simulink model "biomasaCambioEntrada"  (R2018a)
settings: Solver=VariableStepAuto  StartTime=0.0  StopTime=200  RelTol=1e-3
libraries: simulink x3
settings Model: Creator=Asus  LastModifiedBy=Asus
settings CodeAppCC: StateflowObjectComments=on

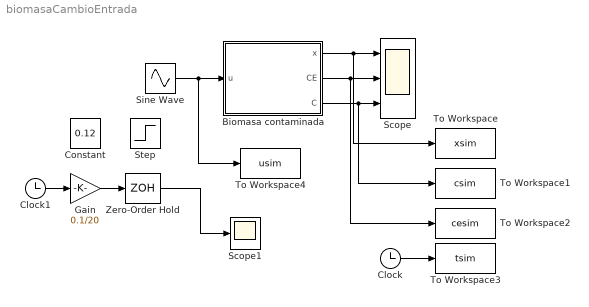
== system biomasaCambioEntrada ==
  Biomasa contaminada : Subsystem  mask(Modelo){par=[0.01,0.01,0.2,0.2,0.1,0.1,5,0.01,2], ci=[2,0,2]}
      mask prompts: par "[n, a, b, h, mu, r0, k0, r1, p]"; ci "[x0, c0, ce0]"
      mask help:
      | Modelo de concentración de contaminación en un ambiente
      | Entrada: contaminación
      | Salidas: biomasa de la población (x), concentración de toxina en el ambiente (Ce), cantidad de toxina en la biomasa de la población (C)
      mask init:
      | n  = par(1);
      | a  = par(2); 
      | b  = par(3);
      | h  = par(4);
      | mu = par(5); 
      | r0 = par(6); 
      | k0 = par(7); 
      | r1 = par(8); 
      | p  = par(9); 
      | x0 = ci(1);
      | c0 = ci(2);
      | ce0 = ci(3);
  Clock : Clock
  Clock1 : Clock
  Constant : Constant  Value=0.12
  Gain : Gain  Gain=0.1/20
  Scope : Scope  NumInputPorts=3
  Scope1 : Scope
  Sine Wave : Sin  Amplitude=0.5  Frequency=0.2  SampleTime=0
  Step : Step  Time=50  After=0.5  SampleTime=0
  To Workspace : ToWorkspace  VariableName=xsim  SampleTime=-1
      settings: Save2DSignal=2-D array (concatenate along first dimension)
  To Workspace1 : ToWorkspace  VariableName=csim  SampleTime=-1
      settings: Save2DSignal=2-D array (concatenate along first dimension)
  To Workspace2 : ToWorkspace  VariableName=cesim  SampleTime=-1
      settings: Save2DSignal=2-D array (concatenate along first dimension)
  To Workspace3 : ToWorkspace  VariableName=tsim  SampleTime=-1
  To Workspace4 : ToWorkspace  VariableName=usim  SampleTime=-1
  Zero-Order Hold : ZeroOrderHold  SampleTime=20
  wires:
  Biomasa contaminada/1(x) -> To Workspace/1, Scope/1
  Clock/1 -> To Workspace3/1
  Biomasa contaminada/2(CE) -> To Workspace2/1, Scope/2
  Biomasa contaminada/3(C) -> To Workspace1/1, Scope/3
  Gain/1 -> Zero-Order Hold/1
  Zero-Order Hold/1 -> Scope1/1
  Clock1/1 -> Gain/1
  Sine Wave/1 -> To Workspace4/1, Biomasa contaminada/1(u)

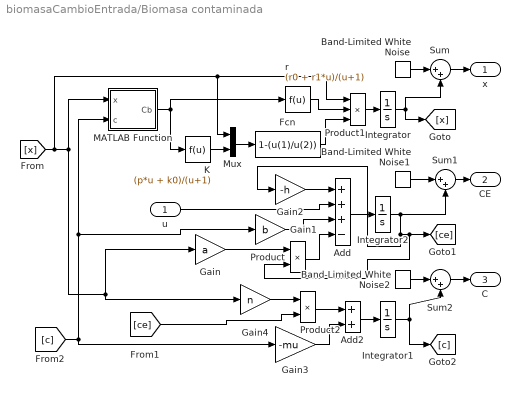
== system biomasaCambioEntrada/Biomasa contaminada ==
  u : Inport
  Add : Sum  Inputs=+++-
  Add2 : Sum
  Band-Limited White Noise : simulink/Sources/Band-Limited White Noise  Cov=0.001  Ts=0.1  seed=[1542869]
  Band-Limited White Noise1 : simulink/Sources/Band-Limited White Noise  Cov=0.001  Ts=0.1  seed=[4785963]
  Band-Limited White Noise2 : simulink/Sources/Band-Limited White Noise  Cov=0.001  Ts=0.1  seed=[5468953]
  Fcn : Fcn  Expr=1-(u(1)/u(2))
  Gain : Gain  Gain=a
  Gain1 : Gain  Gain=b
  Gain2 : Gain  Gain=-h
  Gain3 : Gain  Gain=-mu
  Gain4 : Gain  Gain=n
  Integrator : Integrator  InitialCondition=x0
  Integrator1 : Integrator  InitialCondition=c0
  Integrator2 : Integrator  InitialCondition=ce0
  "K " : Fcn  Expr=(p*u + k0)/(u+1)
  MATLAB Function : MATLAB Function  TreatAsAtomicUnit=on
  Mux : Mux  Inputs=2
  Product : Product
  Product1 : Product  Inputs=3
  Product2 : Product
  Sum : Sum  Inputs=|++
  Sum1 : Sum  Inputs=|++
  Sum2 : Sum  Inputs=|++
  "r " : Fcn  Expr=(r0 + r1*u)/(u+1)
  x : Outport
  CE : Outport  Port=2
  C : Outport  Port=3
  wires:
  Product/1 -> Add/4
  Gain1/1 -> Add/3
  Product1/1 -> Integrator/1
  Mux/1 -> Fcn/1
  u/1 -> Add/2
  Gain2/1 -> Add/1
  Add/1 -> Integrator2/1
  MATLAB Function/1(Cb) -> "r "/1, "K "/1
  "r "/1 -> Product1/2
  Integrator/1 -> Sum/2, [x]
  Fcn/1 -> Product1/3
  [x] -> Mux/1, Product1/1, MATLAB Function/1(x), Gain4/1, Gain/1
  [c] -> Gain1/1, MATLAB Function/2(c), Gain3/1
  [ce] -> Product2/2
  Gain4/1 -> Product2/1
  Product2/1 -> Add2/1
  Gain3/1 -> Add2/2
  Add2/1 -> Integrator1/1
  Integrator1/1 -> Sum2/2, [c]
  Gain/1 -> Product/1
  "K "/1 -> Mux/2
  Sum/1 -> x/1
  Band-Limited White Noise/1 -> Sum/1
  Band-Limited White Noise1/1 -> Sum1/1
  Sum1/1 -> CE/1
  Integrator2/1 -> Gain2/1, Product/2, [ce], Sum1/2
  Band-Limited White Noise2/1 -> Sum2/1
  Sum2/1 -> C/1

== matlab function biomasaCambioEntrada/Biomasa contaminada/MATLAB Function ==
  data: x input; c input; Cb output
function Cb = fcn(x, c)
if x == 0
    Cb = 0;
else
    Cb = c/x;
end
end
